simulink model "parity_error"  (R2017a)
settings: Solver=VariableStepAuto  StartTime=0.0  StopTime=10.0  RelTol=1e-3
settings Model: Creator=joaomanito  LastModifiedBy=joaomanito

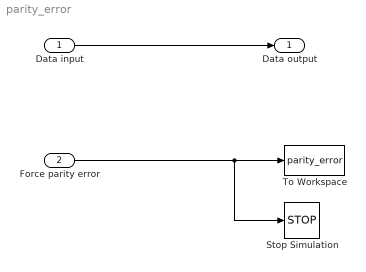
== system parity_error ==
  Data input : Inport
  Force parity error : Inport  Port=2
  Stop Simulation : Stop
  To Workspace : ToWorkspace  VariableName=parity_error  SaveFormat=Timeseries  SampleTime=-1
  Data output : Outport
  wires:
  Force parity error/1 -> Stop Simulation/1, To Workspace/1
  Data input/1 -> Data output/1
